simulink model "foucaultBus"  (R2022b)
settings: Solver=ode23t  StartTime=0.0  StopTime=3600  FixedStep=.1  RelTol=1e-5  EnableMultiTasking=on
PreLoadFcn:
  | % Parameters
  | L = 67;             % Pendulum length [m]
  | g = 9.81;           % Gravitational acceleration [m/s^2]
  | Omega = 2*pi/86400; % Earth's angular velocity of rotation about its axis [rad/sec]
  | lambda = 49/180*pi; % latitude [rad]
  | initial_x = L/100;  % initial x coordinate [m]
  | initial_y = 0;      % initial y coordinate [m]
  | initial_xdot = 0;   % initial x velocity [m/sec]
  | initial_ydot = 0;   % initial y velocity [m/sec]
CloseFcn:
  | close(findobj('Tag','CloseMe'));
settings Model: Creator=The MathWorks Inc.  LastModifiedBy=bensweet
settings SolverCC: AlgebraicLoopSolver=TrustRegion
settings DataIOCC: SaveFormat=StructureWithTime  SaveOutput=off  SaveTime=off  ReturnWorkspaceOutputs=off  SignalLoggingName=sldemo_foucault_output
settings OptimizationCC: ExpressionDepthLimit=2147483647  InitFltsAndDblsToZero=on  LifeSpan=inf
settings DebuggingCC: UnconnectedInputMsg=warning  UnconnectedOutputMsg=warning  UnconnectedLineMsg=warning  PregeneratedLibrarySubsystemCodeDiagnostic=none  SFMachineParentedDataDiag=warning
settings HardwareCC: ProdBitPerPointer=32  ProdBitPerSizeT=32  ProdBitPerPtrDiffT=32  ProdLargestAtomicFloat=None  ProdIntDivRoundTo=Undefined  ProdEndianess=Unspecified  ProdWordSize=32  ProdHWDeviceType=32-bit Generic
settings ModelReferenceCC: EnableRefExpFcnMdlSchedulingChecks=on  PropagateSignalLabelsOutOfModel=off
settings SFSimCC: SimUseLocalCustomCode=off
settings RTWCC: RTWUseLocalCustomCode=off  DLArmComputeVersion=19.05
settings CodeAppCC: StateflowObjectComments=on
settings GRTTargetCC: TargetFcnLib=ansi_tfl_tmw.mat  TargetLangStandard=C89/C90 (ANSI)  CombineOutputUpdateFcns=off  GRTInterface=on
settings ConfigComp: CovMetricSettings=dw  CovSaveCumulativeToWorkspaceVar=on  CovSaveSingleToWorkspaceVar=on  CovExternalEMLEnable=off  CovSFcnEnable=off

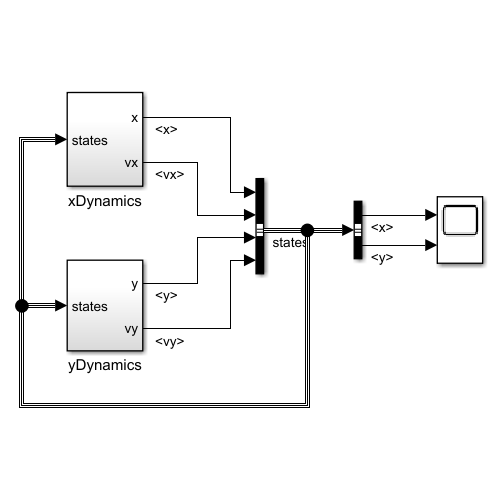
[thumbnail: Simulink's stored preview of the top-level diagram]
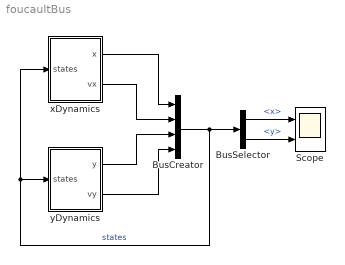
== system foucaultBus ==
  BusCreator : BusCreator  Inputs=4
  BusSelector : BusSelector  OutputSignals=x,y
  Scope : Scope  NumInputPorts=2
  xDynamics : Subsystem
  yDynamics : Subsystem
  wires:
  xDynamics/1(x) -> BusCreator/1
  xDynamics/2(vx) -> BusCreator/2
  yDynamics/1(y) -> BusCreator/3
  yDynamics/2(vy) -> BusCreator/4
  BusCreator/1 -> BusSelector/1, yDynamics/1(states), xDynamics/1(states)  "states"
  BusSelector/1 -> Scope/1  "<x>"
  BusSelector/2 -> Scope/2  "<y>"

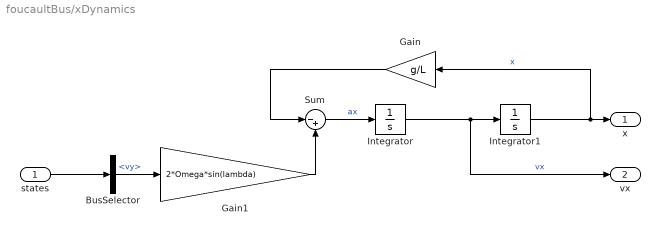
== system foucaultBus/xDynamics ==
  states : Inport
  BusSelector : BusSelector  OutputSignals=vy
  Gain : Gain  Gain=g/L
  Gain1 : Gain  Gain=2*Omega*sin(lambda)
  Integrator : Integrator  InitialCondition=initial_xdot
  Integrator1 : Integrator  InitialCondition=initial_x
  Sum : Sum  Inputs=|-+
  x : Outport  VectorParamsAs1DForOutWhenUnconnected=off
  vx : Outport  Port=2  VectorParamsAs1DForOutWhenUnconnected=off
  wires:
  Integrator/1 -> Integrator1/1, vx/1  "vx"
  Integrator1/1 -> Gain/1, x/1  "x"
  Sum/1 -> Integrator/1  "ax"
  Gain/1 -> Sum/1
  Gain1/1 -> Sum/2
  states/1 -> BusSelector/1
  BusSelector/1 -> Gain1/1  "<vy>"

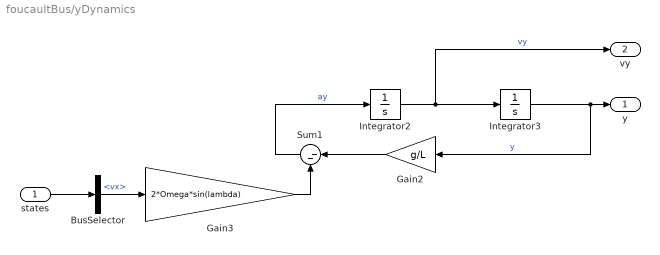
== system foucaultBus/yDynamics ==
  states : Inport
  BusSelector : BusSelector  OutputSignals=vx
  Gain2 : Gain  Gain=g/L
  Gain3 : Gain  Gain=2*Omega*sin(lambda)
  Integrator2 : Integrator  InitialCondition=initial_ydot
  Integrator3 : Integrator  InitialCondition=initial_y
  Sum1 : Sum  Inputs=|--
  y : Outport  VectorParamsAs1DForOutWhenUnconnected=off
  vy : Outport  Port=2  VectorParamsAs1DForOutWhenUnconnected=off
  wires:
  Integrator2/1 -> Integrator3/1, vy/1  "vy"
  Gain2/1 -> Sum1/1
  Gain3/1 -> Sum1/2
  Sum1/1 -> Integrator2/1  "ay"
  Integrator3/1 -> Gain2/1, y/1  "y"
  states/1 -> BusSelector/1
  BusSelector/1 -> Gain3/1  "<vx>"
